simulink model "UPQC_model"  (R2020b)
settings: Solver=FixedStepAuto  StartTime=0.0  StopTime=Tsim  FixedStep=Tsample  MaxStep=Tsample  RelTol=1e-3
values from neighbouring files (symbols this model uses):
  C_parallel_Series = zeros(1,4)    [Netzmodell_Ini_DL.m]    (also in workspace_Ini.mat = [1e-05 1e-05 1e-05 0])
  C_parallel_Shunt = zeros(1,4)    [Netzmodell_Ini_DL.m]    (also in workspace_Ini.mat = [1e-05 1e-05 1e-05 0])
  CC_Ki = 5    [Netzmodell_Ini_DL.m]    (also in workspace_Ini.mat)
  CC_Ki_geg = 5    [Netzmodell_Ini_DL.m]    (also in workspace_Ini.mat)
  CC_Kp = 10    [Netzmodell_Ini_DL.m]    (also in workspace_Ini.mat)
  CC_Kp_geg = 10    [Netzmodell_Ini_DL.m]    (also in workspace_Ini.mat)
  CC_OS =     [workspace_Ini.mat]
  Czk = Szenario.Czk*u    [Netzmodell_Ini_DL.m]    (also in workspace_Ini.mat = 0.003)
  fak_RVC = Szenario.fak_RVC    [Netzmodell_Ini_DL.m]    (also in workspace_Ini.mat = [1 1 1])
  fak_Uns = [1; 1; 1]    [Netzmodell_Ini_DL.m]    (also in workspace_Ini.mat = [1 1 1])
  Flicker_Schaltzeitpunkte_L1 = Schaltzeitpunkte(1,:)    [Netzmodell_Ini_DL.m]    (also in workspace_Ini.mat = 10.5)
  Flicker_Schaltzeitpunkte_L2 = Schaltzeitpunkte(2,:)    [Netzmodell_Ini_DL.m]    (also in workspace_Ini.mat = 10.5)
  Flicker_Schaltzeitpunkte_L3 = Schaltzeitpunkte(3,:)    [Netzmodell_Ini_DL.m]    (also in workspace_Ini.mat = 10.5)
  fs = [f_nom; f_nom; f_nom]    [Netzmodell_Ini_DL.m]    (also in workspace_Ini.mat = [50 50 50])
  fsw = Szenario.fsw*k    [Netzmodell_Ini_DL.m]    (also in workspace_Ini.mat = 20000)
  I_Basis_Ober_L1 = I_Basis_Ober(1)    [Netzmodell_Ini_DL.m]    (also in workspace_Ini.mat = 0)
  I_Basis_Ober_L2 = I_Basis_Ober(2)    [Netzmodell_Ini_DL.m]    (also in workspace_Ini.mat = 0)
  I_Basis_Ober_L3 = I_Basis_Ober(3)    [Netzmodell_Ini_DL.m]    (also in workspace_Ini.mat = 0)
  I_relativ_Ober_L1 = Szenario.I_relativ_Ober_L1    [Netzmodell_Ini_DL.m]    (also in workspace_Ini.mat = [0 100 0 100 100 0 100 100 0 0 0 0 ... (50 elements, 1x50)])
  I_relativ_Ober_L2 = Szenario.I_relativ_Ober_L2    [Netzmodell_Ini_DL.m]    (also in workspace_Ini.mat = [0 100 0 100 100 0 100 100 0 0 0 0 ... (50 elements, 1x50)])
  I_relativ_Ober_L3 = Szenario.I_relativ_Ober_L3    [Netzmodell_Ini_DL.m]    (also in workspace_Ini.mat = [0 100 0 100 100 0 100 100 0 0 0 0 ... (50 elements, 1x50)])
  L_Ausgang_Series = zeros(1,4)    [Netzmodell_Ini_DL.m]    (also in workspace_Ini.mat = [0.00093 0.00093 0.00093 0.00093])
  L_Ausgang_Shunt = zeros(1,4)    [Netzmodell_Ini_DL.m]    (also in workspace_Ini.mat = [0.00093 0.00093 0.00093 0.00093])
  L_Eingang_Series = zeros(1,4)    [Netzmodell_Ini_DL.m]    (also in workspace_Ini.mat = [0.00085 0.00085 0.00085 0.00085])
  L_Eingang_Shunt = zeros(1,4)    [Netzmodell_Ini_DL.m]    (also in workspace_Ini.mat = [0.00085 0.00085 0.00085 0.00085])
  Ls_in = 52.2*u/10    (= 5.22e-06)    [Netzmodell_Ini_DL.m]    (also in workspace_Ini.mat)
  Ltrans = Szenario.Ltrans*m    [Netzmodell_Ini_DL.m]    (also in workspace_Ini.mat = 0.000256)
  OS_off = 6    [Netzmodell_Ini_DL.m]    (also in workspace_Ini.mat)
  OS_on = 1    [Netzmodell_Ini_DL.m]    (also in workspace_Ini.mat)
  Phi_Ober_L1 = Phi_Ober(1)    [Netzmodell_Ini_DL.m]    (also in workspace_Ini.mat = 0)
  Phi_Ober_L2 = Phi_Ober(2)    [Netzmodell_Ini_DL.m]    (also in workspace_Ini.mat = -120)
  Phi_Ober_L3 = Phi_Ober(3)    [Netzmodell_Ini_DL.m]    (also in workspace_Ini.mat = 120)
  Phis = [0; -120; 120]    [Netzmodell_Ini_DL.m]    (also in workspace_Ini.mat = [0 -120 120])
  Pl_Flicker = Pl_Flicker*k    [Netzmodell_Ini_DL.m]    (also in workspace_Ini.mat = [5000 5000 5000])
  Pl_Grund = Szenario.Pl_Grund *k    [Netzmodell_Ini_DL.m]    (also in workspace_Ini.mat = [5 5 5])
  Pl_RVC = Pl_RVC*k    [Netzmodell_Ini_DL.m]    (also in workspace_Ini.mat = [10000 10000 10000])
  Pl_Uns = Pl_Uns*k    [Netzmodell_Ini_DL.m]    (also in workspace_Ini.mat = [25000 10 10])
  Ql_ind_Flicker = Ql_ind_Flicker*k    [Netzmodell_Ini_DL.m]    (also in workspace_Ini.mat = [0 0 0])
  Ql_ind_Grund = Szenario.Ql_ind_Grund*k    [Netzmodell_Ini_DL.m]    (also in workspace_Ini.mat = [0 0 0])
  Ql_ind_RVC = Szenario.Ql_ind_RVC*k    [Netzmodell_Ini_DL.m]    (also in workspace_Ini.mat = [0 0 0])
  Ql_ind_Uns = Ql_ind_Uns*k    [Netzmodell_Ini_DL.m]    (also in workspace_Ini.mat = [0 0 0])
  Ql_kap_Flicker = Ql_kap_Flicker*k    [Netzmodell_Ini_DL.m]    (also in workspace_Ini.mat = [0 0 0])
  Ql_kap_Grund = Szenario.Ql_kap_Grund*k    [Netzmodell_Ini_DL.m]    (also in workspace_Ini.mat = [0 0 0])
  Ql_kap_RVC = Szenario.Ql_kap_RVC*k    [Netzmodell_Ini_DL.m]    (also in workspace_Ini.mat = [0 0 0])
  Ql_kap_Uns = Ql_kap_Uns*k    [Netzmodell_Ini_DL.m]    (also in workspace_Ini.mat = [0 0 0])
  R_Ausgang_Series = zeros(1,4)    [Netzmodell_Ini_DL.m]    (also in workspace_Ini.mat = [0.1 0.1 0.1 0.1])
  R_Ausgang_Shunt = zeros(1,4)    [Netzmodell_Ini_DL.m]    (also in workspace_Ini.mat = [0.1 0.1 0.1 0.1])
  R_Eingang_Series = zeros(1,4)    [Netzmodell_Ini_DL.m]    (also in workspace_Ini.mat = [0.1 0.1 0.1 0.1])
  R_Eingang_Shunt = zeros(1,4)    [Netzmodell_Ini_DL.m]    (also in workspace_Ini.mat = [0.1 0.1 0.1 0.1])
  R_parallel_Series = zeros(1,4)    [Netzmodell_Ini_DL.m]    (also in workspace_Ini.mat = [13 13 13 0])
  R_parallel_Shunt = zeros(1,4)    [Netzmodell_Ini_DL.m]    (also in workspace_Ini.mat = [13 13 13 0])
  R_ZK_Belastung = 20    [Netzmodell_Ini_DL.m]    (also in workspace_Ini.mat)
  Rs_in = 5.2*m/10    (= 0.00052)    [Netzmodell_Ini_DL.m]    (also in workspace_Ini.mat)
  Rtrans = Szenario.Rtrans    [Netzmodell_Ini_DL.m]    (also in workspace_Ini.mat = 0.206)
  RVC_L1_on_off_Zeitpunkte = Szenario.RVC_L1_on_off_Zeitpunkte    [Netzmodell_Ini_DL.m]    (also in workspace_Ini.mat = [10.5 40 10 11 12 13 14 15])
  RVC_L2_on_off_Zeitpunkte = Szenario.RVC_L2_on_off_Zeitpunkte    [Netzmodell_Ini_DL.m]    (also in workspace_Ini.mat = [10.5 40 10 11 12 13 14 15])
  RVC_L3_on_off_Zeitpunkte = Szenario.RVC_L3_on_off_Zeitpunkte    [Netzmodell_Ini_DL.m]    (also in workspace_Ini.mat = [10.5 40 10 11 12 13 14 15])
  RVC_off = 20.5    [Netzmodell_Ini_DL.m]    (also in workspace_Ini.mat)
  RVC_on = 20    [Netzmodell_Ini_DL.m]    (also in workspace_Ini.mat)
  RVC_val = [0.8,0.8,0.8]    [Netzmodell_Ini_DL.m]    (also in workspace_Ini.mat = [0.8 0.8 0.8])
  strans = Szenario.strans    [Netzmodell_Ini_DL.m]    (also in workspace_Ini.mat = 0.25)
  t_breaker_series = tacts    [Netzmodell_Ini_DL.m]    (also in workspace_Ini.mat = 0.5)
  tact = Szenario.tact    [Netzmodell_Ini_DL.m]    (also in workspace_Ini.mat = 0.5)
  tact_OS_Regler = Szenario.tact_OS_Regler    [Netzmodell_Ini_DL.m]    (also in workspace_Ini.mat = 0.5)
  tact_QU = 10    [Netzmodell_Ini_DL.m]    (also in workspace_Ini.mat)
  tacts = Szenario.tacts    [Netzmodell_Ini_DL.m]    (also in workspace_Ini.mat = 0.5)
  Tsample = Szenario.Tsample    [Netzmodell_Ini_DL.m]    (also in workspace_Ini.mat = 5e-06)
  Uns_L1_on_off_Zeitpunkte = Szenario.Uns_L1_on_off_Zeitpunkte    [Netzmodell_Ini_DL.m]    (also in workspace_Ini.mat = [1 6 10 11 12 13 14 15])
  Uns_L2_on_off_Zeitpunkte = Szenario.Uns_L2_on_off_Zeitpunkte    [Netzmodell_Ini_DL.m]    (also in workspace_Ini.mat = [10 30 10 11 12 13 14 15])
  Uns_L3_on_off_Zeitpunkte = Szenario.Uns_L3_on_off_Zeitpunkte    [Netzmodell_Ini_DL.m]    (also in workspace_Ini.mat = [10 30 10 11 12 13 14 15])
  Us = [Us_Amp; Us_Amp; Us_Amp]    [Netzmodell_Ini_DL.m]    (also in workspace_Ini.mat = [326.598632371 326.598632371 326.598632371])
  Us_Amp = sqrt(2)*400/sqrt(3)    [Netzmodell_Ini_DL.m]    (also in workspace_Ini.mat = 326.598632371)
  VC_Ki_gegen = 30    [Netzmodell_Ini_DL.m]    (also in workspace_Ini.mat)
  VC_Ki_gegen_shunt = 15    [Netzmodell_Ini_DL.m]    (also in workspace_Ini.mat)
  VC_Ki_mit = 5    [Netzmodell_Ini_DL.m]    (also in workspace_Ini.mat)
  VC_Kp_gegen = 5    [workspace_Ini.mat]
  VC_Kp_gegen_shunt = 2    [Netzmodell_Ini_DL.m]    (also in workspace_Ini.mat)
  VC_Kp_mit = 10    [Netzmodell_Ini_DL.m]    (also in workspace_Ini.mat)
  VC_ZK_Ki = 5    [Netzmodell_Ini_DL.m]    (also in workspace_Ini.mat)
  VC_ZK_Kp = 0.5    [Netzmodell_Ini_DL.m]    (also in workspace_Ini.mat)
  Vielfache_Ober_L1 = Szenario.Vielfache_Ober_L1    [Netzmodell_Ini_DL.m]    (also in workspace_Ini.mat = [1 2 3 4 5 6 7 8 9 10 11 12 ... (50 elements, 1x50)])
  Vielfache_Ober_L2 = Szenario.Vielfache_Ober_L2    [Netzmodell_Ini_DL.m]    (also in workspace_Ini.mat = [1 2 3 4 5 6 7 8 9 10 11 12 ... (50 elements, 1x50)])
  Vielfache_Ober_L3 = Szenario.Vielfache_Ober_L3    [Netzmodell_Ini_DL.m]    (also in workspace_Ini.mat = [1 2 3 4 5 6 7 8 9 10 11 12 ... (50 elements, 1x50)])
  ZK_Belastung_off = 100    [Netzmodell_Ini_DL.m]    (also in workspace_Ini.mat)
  ZK_Belastung_on = 100    [Netzmodell_Ini_DL.m]    (also in workspace_Ini.mat)
  Zwischenkreisspannung = 700    [Netzmodell_Ini_DL.m]    (also in workspace_Ini.mat)
undefined symbols (not defined in the file or in its folder): LAusgang, RReiheL3
libraries: powerlib x221, powerlib_meascontrol x80, pid_lib x23, eeTransforms x4, eePwmGeneratorTwoLevel x2, dspstat3 x1
(part 8 of 16)

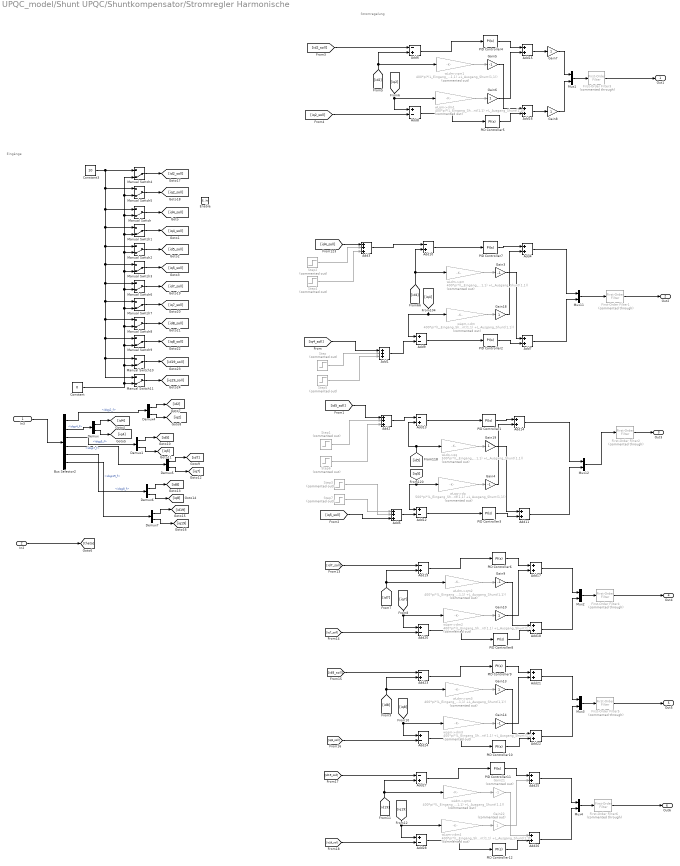
== system UPQC_model/Shunt UPQC/Shuntkompensator/Stromregler Harmonische ==
  note: Eingänge
  note: Stromregelung
  In3 : Inport
  In2 : Inport  Port=2
  Enable : EnablePort
  Add{1..3,5} (4 alike) : Sum  Inputs=+++
  Add{6,10,13,19,23,27} (6 alike) : Sum  Inputs=-+
  Add{4,7,11,14..18,21..22,25..26} (12 alike) : Sum
  Add{8..9,12,20,24,28} (6 alike) : Sum  Inputs=+-
  Bus Selector2 : BusSelector  OutputSignals=idqg2_f,idqp4_f,idqg5_f,idqp7_f,idqg8_f,idqp19_f
  Constant : Constant  Value=0
  Constant3 : Constant  Value=10
  Demux{,1,4..7} (6 alike) : Demux  Outputs=2
  First-Order Filter{1..6} (6 alike) : powerlib_meascontrol/Filters/First-Order Filter  Commented=through  FilterType=Lowpass  Tc=1/(2*25*pi/sqrt(2))  Ts=0  Initialize=off  Vac_Init=[0, 0, 60]  Vdc_Init=0  PlotResponse=off  FreqRange="[0,  30,  1]"
  Gain{6..8,10,13,18..19} (7 alike) : Gain
  Gain{3..5,9,14} (5 alike) : Gain  Gain=-1
  Gain21 : Gain  Commented=on  Gain=-1
  Gain22 : Gain  Commented=on
  Manual Switch{,1..11} (12 alike) : ManualSwitch  CurrentSetting=0
  Mux{1..4,11..12} (6 alike) : Mux  Inputs=2
  PID Controller1 : pid_lib/PID Controller  Controller=PI  Form=Parallel  TimeDomain=Continuous-time  UseExternalTs=off  SampleTime=-1  IntegratorMethod=Forward Euler  FilterMethod=Forward Euler  ControllerParametersSource=internal  P=CC_OS.Kp5  I=CC_OS.Ki5  D=0  UseFilter=on  N=100  TunerSelectOption=Transfer Function Based (PID Tuner App)  InitialConditionSource=internal  InitialConditionForIntegrator=0  InitialConditionForFilter=0  DifferentiatorICPrevScaledInput=0  ExternalReset=none  TrackingMode=off  Kt=1  LimitOutput=off  SatLimitsSource=internal  UpperSaturationLimit=800  LowerSaturationLimit=-800  LinearizeAsGain=on  AntiWindupMode=none  Kb=1  POutMin=[]  POutMax=[]  IOutMin=[]  IOutMax=[]  DOutMin=[]  DOutMax=[]  NOutMin=[]  NOutMax=[]  SumOutMin=[]  SumOutMax=[]  SaturationOutMin=[]  SaturationOutMax=[]  PParamMin=[]  PParamMax=[]  IParamMin=[]  IParamMax=[]  DParamMin=[]  DParamMax=[]  NParamMin=[]  NParamMax=[]  KbParamMin=[]  KbParamMax=[]  KtParamMin=[]  KtParamMax=[]  KbOutMin=[]  KbOutMax=[]  KtOutMin=[]  KtOutMax=[]  IntegratorOutMin=[]  IntegratorOutMax=[]  FilterOutMin=[]  FilterOutMax=[]  SumI1OutMin=[]  SumI1OutMax=[]  SumI2OutMin=[]  SumI2OutMax=[]  SumI3OutMin=[]  SumI3OutMax=[]  SumI4OutMin=[]  SumI4OutMax=[]  SumDOutMin=[]  SumDOutMax=[]  DifferentiatorOutMin=[]  DifferentiatorOutMax=[]  FilterDiffOutCoefMin=[]  FilterDiffOutCoefMax=[]  ReciprocalOutMin=[]  ReciprocalOutMax=[]  SumDenOutMin=[]  SumDenOutMax=[]  SumNumOutMin=[]  SumNumOutMax=[]  DivideOutMin=[]  DivideOutMax=[]  UdiffTsProdOutMin=[]  UdiffTsProdOutMax=[]  NTsProdOutMin=[]  NTsProdOutMax=[]  UintegralTsProdOutMin=[]  UintegralTsProdOutMax=[]  UngainTsProdOutMin=[]  UngainTsProdOutMax=[]  IntegratorContinuousStateAttributes=''  IntegratorStateMustResolveToSignalObject=off  IntegratorRTWStateStorageClass=Auto  FilterContinuousStateAttributes=''  FilterStateMustResolveToSignalObject=off  FilterRTWStateStorageClass=Auto  ParallelPVariant=InternalParameters  IdealPVariant=Disabled  IVariant=InternalParameters  DVariant=Disabled  IntegratorVariant=Continuous  SatVariant=Disabled  AWVariant=Passthrough  PCopyVariant=Disabled  TRVariant=Disabled  FdbkBlocksVariant=Forward  IdealPFdbkVariant=Disabled  SatFdbkVariant=Disabled  DerivativeFilterVariant=Disabled  NVariant=Disabled  NCopyVariant=Disabled_SignalSpec  FilterICVariant=Disabled  IntegratorICVariant=InternalICs  ExternalResetVariant=Disabled  TRSumVariant=Passthrough  SumFdbkVariant=Disabled  SumVariant=Sum_PI  TsampFilterVariant=InternalTs  TsampNgainVariant=Passthrough  TsampIntegralVariant=Passthrough  ExternalSaturationOutDataTypeStr=Inherit: Same as second input
  PID Controller10 : pid_lib/PID Controller  Controller=PI  Form=Parallel  TimeDomain=Continuous-time  UseExternalTs=off  SampleTime=-1  IntegratorMethod=Forward Euler  FilterMethod=Forward Euler  ControllerParametersSource=internal  P=CC_OS.Kp8  I=CC_OS.Ki8  D=0  UseFilter=on  N=100  TunerSelectOption=Transfer Function Based (PID Tuner App)  InitialConditionSource=internal  InitialConditionForIntegrator=0  InitialConditionForFilter=0  DifferentiatorICPrevScaledInput=0  ExternalReset=none  TrackingMode=off  Kt=1  LimitOutput=off  SatLimitsSource=internal  UpperSaturationLimit=800  LowerSaturationLimit=-800  LinearizeAsGain=on  AntiWindupMode=none  Kb=1  POutMin=[]  POutMax=[]  IOutMin=[]  IOutMax=[]  DOutMin=[]  DOutMax=[]  NOutMin=[]  NOutMax=[]  SumOutMin=[]  SumOutMax=[]  SaturationOutMin=[]  SaturationOutMax=[]  PParamMin=[]  PParamMax=[]  IParamMin=[]  IParamMax=[]  DParamMin=[]  DParamMax=[]  NParamMin=[]  NParamMax=[]  KbParamMin=[]  KbParamMax=[]  KtParamMin=[]  KtParamMax=[]  KbOutMin=[]  KbOutMax=[]  KtOutMin=[]  KtOutMax=[]  IntegratorOutMin=[]  IntegratorOutMax=[]  FilterOutMin=[]  FilterOutMax=[]  SumI1OutMin=[]  SumI1OutMax=[]  SumI2OutMin=[]  SumI2OutMax=[]  SumI3OutMin=[]  SumI3OutMax=[]  SumI4OutMin=[]  SumI4OutMax=[]  SumDOutMin=[]  SumDOutMax=[]  DifferentiatorOutMin=[]  DifferentiatorOutMax=[]  FilterDiffOutCoefMin=[]  FilterDiffOutCoefMax=[]  ReciprocalOutMin=[]  ReciprocalOutMax=[]  SumDenOutMin=[]  SumDenOutMax=[]  SumNumOutMin=[]  SumNumOutMax=[]  DivideOutMin=[]  DivideOutMax=[]  UdiffTsProdOutMin=[]  UdiffTsProdOutMax=[]  NTsProdOutMin=[]  NTsProdOutMax=[]  UintegralTsProdOutMin=[]  UintegralTsProdOutMax=[]  UngainTsProdOutMin=[]  UngainTsProdOutMax=[]  IntegratorContinuousStateAttributes=''  IntegratorStateMustResolveToSignalObject=off  IntegratorRTWStateStorageClass=Auto  FilterContinuousStateAttributes=''  FilterStateMustResolveToSignalObject=off  FilterRTWStateStorageClass=Auto  ParallelPVariant=InternalParameters  IdealPVariant=Disabled  IVariant=InternalParameters  DVariant=Disabled  IntegratorVariant=Continuous  SatVariant=Disabled  AWVariant=Passthrough  PCopyVariant=Disabled  TRVariant=Disabled  FdbkBlocksVariant=Forward  IdealPFdbkVariant=Disabled  SatFdbkVariant=Disabled  DerivativeFilterVariant=Disabled  NVariant=Disabled  NCopyVariant=Disabled_SignalSpec  FilterICVariant=Disabled  IntegratorICVariant=InternalICs  ExternalResetVariant=Disabled  TRSumVariant=Passthrough  SumFdbkVariant=Disabled  SumVariant=Sum_PI  TsampFilterVariant=InternalTs  TsampNgainVariant=Passthrough  TsampIntegralVariant=Passthrough  ExternalSaturationOutDataTypeStr=Inherit: Same as second input
  PID Controller11 : pid_lib/PID Controller  Controller=PI  Form=Parallel  TimeDomain=Continuous-time  UseExternalTs=off  SampleTime=-1  IntegratorMethod=Forward Euler  FilterMethod=Forward Euler  ControllerParametersSource=internal  P=CC_OS.Kp19  I=CC_OS.Ki19  D=0  UseFilter=on  N=100  TunerSelectOption=Transfer Function Based (PID Tuner App)  InitialConditionSource=internal  InitialConditionForIntegrator=0  InitialConditionForFilter=0  DifferentiatorICPrevScaledInput=0  ExternalReset=none  TrackingMode=off  Kt=1  LimitOutput=off  SatLimitsSource=internal  UpperSaturationLimit=800  LowerSaturationLimit=-800  LinearizeAsGain=on  AntiWindupMode=none  Kb=1  POutMin=[]  POutMax=[]  IOutMin=[]  IOutMax=[]  DOutMin=[]  DOutMax=[]  NOutMin=[]  NOutMax=[]  SumOutMin=[]  SumOutMax=[]  SaturationOutMin=[]  SaturationOutMax=[]  PParamMin=[]  PParamMax=[]  IParamMin=[]  IParamMax=[]  DParamMin=[]  DParamMax=[]  NParamMin=[]  NParamMax=[]  KbParamMin=[]  KbParamMax=[]  KtParamMin=[]  KtParamMax=[]  KbOutMin=[]  KbOutMax=[]  KtOutMin=[]  KtOutMax=[]  IntegratorOutMin=[]  IntegratorOutMax=[]  FilterOutMin=[]  FilterOutMax=[]  SumI1OutMin=[]  SumI1OutMax=[]  SumI2OutMin=[]  SumI2OutMax=[]  SumI3OutMin=[]  SumI3OutMax=[]  SumI4OutMin=[]  SumI4OutMax=[]  SumDOutMin=[]  SumDOutMax=[]  DifferentiatorOutMin=[]  DifferentiatorOutMax=[]  FilterDiffOutCoefMin=[]  FilterDiffOutCoefMax=[]  ReciprocalOutMin=[]  ReciprocalOutMax=[]  SumDenOutMin=[]  SumDenOutMax=[]  SumNumOutMin=[]  SumNumOutMax=[]  DivideOutMin=[]  DivideOutMax=[]  UdiffTsProdOutMin=[]  UdiffTsProdOutMax=[]  NTsProdOutMin=[]  NTsProdOutMax=[]  UintegralTsProdOutMin=[]  UintegralTsProdOutMax=[]  UngainTsProdOutMin=[]  UngainTsProdOutMax=[]  IntegratorContinuousStateAttributes=''  IntegratorStateMustResolveToSignalObject=off  IntegratorRTWStateStorageClass=Auto  FilterContinuousStateAttributes=''  FilterStateMustResolveToSignalObject=off  FilterRTWStateStorageClass=Auto  ParallelPVariant=InternalParameters  IdealPVariant=Disabled  IVariant=InternalParameters  DVariant=Disabled  IntegratorVariant=Continuous  SatVariant=Disabled  AWVariant=Passthrough  PCopyVariant=Disabled  TRVariant=Disabled  FdbkBlocksVariant=Forward  IdealPFdbkVariant=Disabled  SatFdbkVariant=Disabled  DerivativeFilterVariant=Disabled  NVariant=Disabled  NCopyVariant=Disabled_SignalSpec  FilterICVariant=Disabled  IntegratorICVariant=InternalICs  ExternalResetVariant=Disabled  TRSumVariant=Passthrough  SumFdbkVariant=Disabled  SumVariant=Sum_PI  TsampFilterVariant=InternalTs  TsampNgainVariant=Passthrough  TsampIntegralVariant=Passthrough  ExternalSaturationOutDataTypeStr=Inherit: Same as second input
  PID Controller12 : pid_lib/PID Controller  Controller=PI  Form=Parallel  TimeDomain=Continuous-time  UseExternalTs=off  SampleTime=-1  IntegratorMethod=Forward Euler  FilterMethod=Forward Euler  ControllerParametersSource=internal  P=CC_OS.Kp19  I=CC_OS.Ki19  D=0  UseFilter=on  N=100  TunerSelectOption=Transfer Function Based (PID Tuner App)  InitialConditionSource=internal  InitialConditionForIntegrator=0  InitialConditionForFilter=0  DifferentiatorICPrevScaledInput=0  ExternalReset=none  TrackingMode=off  Kt=1  LimitOutput=off  SatLimitsSource=internal  UpperSaturationLimit=800  LowerSaturationLimit=-800  LinearizeAsGain=on  AntiWindupMode=none  Kb=1  POutMin=[]  POutMax=[]  IOutMin=[]  IOutMax=[]  DOutMin=[]  DOutMax=[]  NOutMin=[]  NOutMax=[]  SumOutMin=[]  SumOutMax=[]  SaturationOutMin=[]  SaturationOutMax=[]  PParamMin=[]  PParamMax=[]  IParamMin=[]  IParamMax=[]  DParamMin=[]  DParamMax=[]  NParamMin=[]  NParamMax=[]  KbParamMin=[]  KbParamMax=[]  KtParamMin=[]  KtParamMax=[]  KbOutMin=[]  KbOutMax=[]  KtOutMin=[]  KtOutMax=[]  IntegratorOutMin=[]  IntegratorOutMax=[]  FilterOutMin=[]  FilterOutMax=[]  SumI1OutMin=[]  SumI1OutMax=[]  SumI2OutMin=[]  SumI2OutMax=[]  SumI3OutMin=[]  SumI3OutMax=[]  SumI4OutMin=[]  SumI4OutMax=[]  SumDOutMin=[]  SumDOutMax=[]  DifferentiatorOutMin=[]  DifferentiatorOutMax=[]  FilterDiffOutCoefMin=[]  FilterDiffOutCoefMax=[]  ReciprocalOutMin=[]  ReciprocalOutMax=[]  SumDenOutMin=[]  SumDenOutMax=[]  SumNumOutMin=[]  SumNumOutMax=[]  DivideOutMin=[]  DivideOutMax=[]  UdiffTsProdOutMin=[]  UdiffTsProdOutMax=[]  NTsProdOutMin=[]  NTsProdOutMax=[]  UintegralTsProdOutMin=[]  UintegralTsProdOutMax=[]  UngainTsProdOutMin=[]  UngainTsProdOutMax=[]  IntegratorContinuousStateAttributes=''  IntegratorStateMustResolveToSignalObject=off  IntegratorRTWStateStorageClass=Auto  FilterContinuousStateAttributes=''  FilterStateMustResolveToSignalObject=off  FilterRTWStateStorageClass=Auto  ParallelPVariant=InternalParameters  IdealPVariant=Disabled  IVariant=InternalParameters  DVariant=Disabled  IntegratorVariant=Continuous  SatVariant=Disabled  AWVariant=Passthrough  PCopyVariant=Disabled  TRVariant=Disabled  FdbkBlocksVariant=Forward  IdealPFdbkVariant=Disabled  SatFdbkVariant=Disabled  DerivativeFilterVariant=Disabled  NVariant=Disabled  NCopyVariant=Disabled_SignalSpec  FilterICVariant=Disabled  IntegratorICVariant=InternalICs  ExternalResetVariant=Disabled  TRSumVariant=Passthrough  SumFdbkVariant=Disabled  SumVariant=Sum_PI  TsampFilterVariant=InternalTs  TsampNgainVariant=Passthrough  TsampIntegralVariant=Passthrough  ExternalSaturationOutDataTypeStr=Inherit: Same as second input
  PID Controller2 : pid_lib/PID Controller  Controller=PI  Form=Parallel  TimeDomain=Continuous-time  UseExternalTs=off  SampleTime=-1  IntegratorMethod=Forward Euler  FilterMethod=Forward Euler  ControllerParametersSource=internal  P=CC_OS.Kp4  I=CC_OS.Ki4  D=0  UseFilter=on  N=100  TunerSelectOption=Transfer Function Based (PID Tuner App)  InitialConditionSource=internal  InitialConditionForIntegrator=0  InitialConditionForFilter=0  DifferentiatorICPrevScaledInput=0  ExternalReset=none  TrackingMode=off  Kt=1  LimitOutput=off  SatLimitsSource=internal  UpperSaturationLimit=800  LowerSaturationLimit=-800  LinearizeAsGain=on  AntiWindupMode=none  Kb=1  POutMin=[]  POutMax=[]  IOutMin=[]  IOutMax=[]  DOutMin=[]  DOutMax=[]  NOutMin=[]  NOutMax=[]  SumOutMin=[]  SumOutMax=[]  SaturationOutMin=[]  SaturationOutMax=[]  PParamMin=[]  PParamMax=[]  IParamMin=[]  IParamMax=[]  DParamMin=[]  DParamMax=[]  NParamMin=[]  NParamMax=[]  KbParamMin=[]  KbParamMax=[]  KtParamMin=[]  KtParamMax=[]  KbOutMin=[]  KbOutMax=[]  KtOutMin=[]  KtOutMax=[]  IntegratorOutMin=[]  IntegratorOutMax=[]  FilterOutMin=[]  FilterOutMax=[]  SumI1OutMin=[]  SumI1OutMax=[]  SumI2OutMin=[]  SumI2OutMax=[]  SumI3OutMin=[]  SumI3OutMax=[]  SumI4OutMin=[]  SumI4OutMax=[]  SumDOutMin=[]  SumDOutMax=[]  DifferentiatorOutMin=[]  DifferentiatorOutMax=[]  FilterDiffOutCoefMin=[]  FilterDiffOutCoefMax=[]  ReciprocalOutMin=[]  ReciprocalOutMax=[]  SumDenOutMin=[]  SumDenOutMax=[]  SumNumOutMin=[]  SumNumOutMax=[]  DivideOutMin=[]  DivideOutMax=[]  UdiffTsProdOutMin=[]  UdiffTsProdOutMax=[]  NTsProdOutMin=[]  NTsProdOutMax=[]  UintegralTsProdOutMin=[]  UintegralTsProdOutMax=[]  UngainTsProdOutMin=[]  UngainTsProdOutMax=[]  IntegratorContinuousStateAttributes=''  IntegratorStateMustResolveToSignalObject=off  IntegratorRTWStateStorageClass=Auto  FilterContinuousStateAttributes=''  FilterStateMustResolveToSignalObject=off  FilterRTWStateStorageClass=Auto  ParallelPVariant=InternalParameters  IdealPVariant=Disabled  IVariant=InternalParameters  DVariant=Disabled  IntegratorVariant=Continuous  SatVariant=Disabled  AWVariant=Passthrough  PCopyVariant=Disabled  TRVariant=Disabled  FdbkBlocksVariant=Forward  IdealPFdbkVariant=Disabled  SatFdbkVariant=Disabled  DerivativeFilterVariant=Disabled  NVariant=Disabled  NCopyVariant=Disabled_SignalSpec  FilterICVariant=Disabled  IntegratorICVariant=InternalICs  ExternalResetVariant=Disabled  TRSumVariant=Passthrough  SumFdbkVariant=Disabled  SumVariant=Sum_PI  TsampFilterVariant=InternalTs  TsampNgainVariant=Passthrough  TsampIntegralVariant=Passthrough  ExternalSaturationOutDataTypeStr=Inherit: Same as second input
  PID Controller3 : pid_lib/PID Controller  Controller=PI  Form=Parallel  TimeDomain=Continuous-time  UseExternalTs=off  SampleTime=-1  IntegratorMethod=Forward Euler  FilterMethod=Forward Euler  ControllerParametersSource=internal  P=CC_OS.Kp5  I=CC_OS.Ki5  D=0  UseFilter=on  N=100  TunerSelectOption=Transfer Function Based (PID Tuner App)  InitialConditionSource=internal  InitialConditionForIntegrator=0  InitialConditionForFilter=0  DifferentiatorICPrevScaledInput=0  ExternalReset=none  TrackingMode=off  Kt=1  LimitOutput=off  SatLimitsSource=internal  UpperSaturationLimit=800  LowerSaturationLimit=-800  LinearizeAsGain=on  AntiWindupMode=none  Kb=1  POutMin=[]  POutMax=[]  IOutMin=[]  IOutMax=[]  DOutMin=[]  DOutMax=[]  NOutMin=[]  NOutMax=[]  SumOutMin=[]  SumOutMax=[]  SaturationOutMin=[]  SaturationOutMax=[]  PParamMin=[]  PParamMax=[]  IParamMin=[]  IParamMax=[]  DParamMin=[]  DParamMax=[]  NParamMin=[]  NParamMax=[]  KbParamMin=[]  KbParamMax=[]  KtParamMin=[]  KtParamMax=[]  KbOutMin=[]  KbOutMax=[]  KtOutMin=[]  KtOutMax=[]  IntegratorOutMin=[]  IntegratorOutMax=[]  FilterOutMin=[]  FilterOutMax=[]  SumI1OutMin=[]  SumI1OutMax=[]  SumI2OutMin=[]  SumI2OutMax=[]  SumI3OutMin=[]  SumI3OutMax=[]  SumI4OutMin=[]  SumI4OutMax=[]  SumDOutMin=[]  SumDOutMax=[]  DifferentiatorOutMin=[]  DifferentiatorOutMax=[]  FilterDiffOutCoefMin=[]  FilterDiffOutCoefMax=[]  ReciprocalOutMin=[]  ReciprocalOutMax=[]  SumDenOutMin=[]  SumDenOutMax=[]  SumNumOutMin=[]  SumNumOutMax=[]  DivideOutMin=[]  DivideOutMax=[]  UdiffTsProdOutMin=[]  UdiffTsProdOutMax=[]  NTsProdOutMin=[]  NTsProdOutMax=[]  UintegralTsProdOutMin=[]  UintegralTsProdOutMax=[]  UngainTsProdOutMin=[]  UngainTsProdOutMax=[]  IntegratorContinuousStateAttributes=''  IntegratorStateMustResolveToSignalObject=off  IntegratorRTWStateStorageClass=Auto  FilterContinuousStateAttributes=''  FilterStateMustResolveToSignalObject=off  FilterRTWStateStorageClass=Auto  ParallelPVariant=InternalParameters  IdealPVariant=Disabled  IVariant=InternalParameters  DVariant=Disabled  IntegratorVariant=Continuous  SatVariant=Disabled  AWVariant=Passthrough  PCopyVariant=Disabled  TRVariant=Disabled  FdbkBlocksVariant=Forward  IdealPFdbkVariant=Disabled  SatFdbkVariant=Disabled  DerivativeFilterVariant=Disabled  NVariant=Disabled  NCopyVariant=Disabled_SignalSpec  FilterICVariant=Disabled  IntegratorICVariant=InternalICs  ExternalResetVariant=Disabled  TRSumVariant=Passthrough  SumFdbkVariant=Disabled  SumVariant=Sum_PI  TsampFilterVariant=InternalTs  TsampNgainVariant=Passthrough  TsampIntegralVariant=Passthrough  ExternalSaturationOutDataTypeStr=Inherit: Same as second input
  PID Controller4 : pid_lib/PID Controller  Controller=PI  Form=Parallel  TimeDomain=Continuous-time  UseExternalTs=off  SampleTime=-1  IntegratorMethod=Forward Euler  FilterMethod=Forward Euler  ControllerParametersSource=internal  P=CC_OS.Kp2  I=CC_OS.Ki2  D=0  UseFilter=on  N=100  TunerSelectOption=Transfer Function Based (PID Tuner App)  InitialConditionSource=internal  InitialConditionForIntegrator=0  InitialConditionForFilter=0  DifferentiatorICPrevScaledInput=0  ExternalReset=none  TrackingMode=off  Kt=1  LimitOutput=off  SatLimitsSource=internal  UpperSaturationLimit=800  LowerSaturationLimit=-800  LinearizeAsGain=on  AntiWindupMode=none  Kb=1  POutMin=[]  POutMax=[]  IOutMin=[]  IOutMax=[]  DOutMin=[]  DOutMax=[]  NOutMin=[]  NOutMax=[]  SumOutMin=[]  SumOutMax=[]  SaturationOutMin=[]  SaturationOutMax=[]  PParamMin=[]  PParamMax=[]  IParamMin=[]  IParamMax=[]  DParamMin=[]  DParamMax=[]  NParamMin=[]  NParamMax=[]  KbParamMin=[]  KbParamMax=[]  KtParamMin=[]  KtParamMax=[]  KbOutMin=[]  KbOutMax=[]  KtOutMin=[]  KtOutMax=[]  IntegratorOutMin=[]  IntegratorOutMax=[]  FilterOutMin=[]  FilterOutMax=[]  SumI1OutMin=[]  SumI1OutMax=[]  SumI2OutMin=[]  SumI2OutMax=[]  SumI3OutMin=[]  SumI3OutMax=[]  SumI4OutMin=[]  SumI4OutMax=[]  SumDOutMin=[]  SumDOutMax=[]  DifferentiatorOutMin=[]  DifferentiatorOutMax=[]  FilterDiffOutCoefMin=[]  FilterDiffOutCoefMax=[]  ReciprocalOutMin=[]  ReciprocalOutMax=[]  SumDenOutMin=[]  SumDenOutMax=[]  SumNumOutMin=[]  SumNumOutMax=[]  DivideOutMin=[]  DivideOutMax=[]  UdiffTsProdOutMin=[]  UdiffTsProdOutMax=[]  NTsProdOutMin=[]  NTsProdOutMax=[]  UintegralTsProdOutMin=[]  UintegralTsProdOutMax=[]  UngainTsProdOutMin=[]  UngainTsProdOutMax=[]  IntegratorContinuousStateAttributes=''  IntegratorStateMustResolveToSignalObject=off  IntegratorRTWStateStorageClass=Auto  FilterContinuousStateAttributes=''  FilterStateMustResolveToSignalObject=off  FilterRTWStateStorageClass=Auto  ParallelPVariant=InternalParameters  IdealPVariant=Disabled  IVariant=InternalParameters  DVariant=Disabled  IntegratorVariant=Continuous  SatVariant=Disabled  AWVariant=Passthrough  PCopyVariant=Disabled  TRVariant=Disabled  FdbkBlocksVariant=Forward  IdealPFdbkVariant=Disabled  SatFdbkVariant=Disabled  DerivativeFilterVariant=Disabled  NVariant=Disabled  NCopyVariant=Disabled_SignalSpec  FilterICVariant=Disabled  IntegratorICVariant=InternalICs  ExternalResetVariant=Disabled  TRSumVariant=Passthrough  SumFdbkVariant=Disabled  SumVariant=Sum_PI  TsampFilterVariant=InternalTs  TsampNgainVariant=Passthrough  TsampIntegralVariant=Passthrough  ExternalSaturationOutDataTypeStr=Inherit: Same as second input
  PID Controller5 : pid_lib/PID Controller  Controller=PI  Form=Parallel  TimeDomain=Continuous-time  UseExternalTs=off  SampleTime=-1  IntegratorMethod=Forward Euler  FilterMethod=Forward Euler  ControllerParametersSource=internal  P=CC_OS.Kp2  I=CC_OS.Ki2  D=0  UseFilter=on  N=100  TunerSelectOption=Transfer Function Based (PID Tuner App)  InitialConditionSource=internal  InitialConditionForIntegrator=0  InitialConditionForFilter=0  DifferentiatorICPrevScaledInput=0  ExternalReset=none  TrackingMode=off  Kt=1  LimitOutput=off  SatLimitsSource=internal  UpperSaturationLimit=800  LowerSaturationLimit=-800  LinearizeAsGain=on  AntiWindupMode=none  Kb=1  POutMin=[]  POutMax=[]  IOutMin=[]  IOutMax=[]  DOutMin=[]  DOutMax=[]  NOutMin=[]  NOutMax=[]  SumOutMin=[]  SumOutMax=[]  SaturationOutMin=[]  SaturationOutMax=[]  PParamMin=[]  PParamMax=[]  IParamMin=[]  IParamMax=[]  DParamMin=[]  DParamMax=[]  NParamMin=[]  NParamMax=[]  KbParamMin=[]  KbParamMax=[]  KtParamMin=[]  KtParamMax=[]  KbOutMin=[]  KbOutMax=[]  KtOutMin=[]  KtOutMax=[]  IntegratorOutMin=[]  IntegratorOutMax=[]  FilterOutMin=[]  FilterOutMax=[]  SumI1OutMin=[]  SumI1OutMax=[]  SumI2OutMin=[]  SumI2OutMax=[]  SumI3OutMin=[]  SumI3OutMax=[]  SumI4OutMin=[]  SumI4OutMax=[]  SumDOutMin=[]  SumDOutMax=[]  DifferentiatorOutMin=[]  DifferentiatorOutMax=[]  FilterDiffOutCoefMin=[]  FilterDiffOutCoefMax=[]  ReciprocalOutMin=[]  ReciprocalOutMax=[]  SumDenOutMin=[]  SumDenOutMax=[]  SumNumOutMin=[]  SumNumOutMax=[]  DivideOutMin=[]  DivideOutMax=[]  UdiffTsProdOutMin=[]  UdiffTsProdOutMax=[]  NTsProdOutMin=[]  NTsProdOutMax=[]  UintegralTsProdOutMin=[]  UintegralTsProdOutMax=[]  UngainTsProdOutMin=[]  UngainTsProdOutMax=[]  IntegratorContinuousStateAttributes=''  IntegratorStateMustResolveToSignalObject=off  IntegratorRTWStateStorageClass=Auto  FilterContinuousStateAttributes=''  FilterStateMustResolveToSignalObject=off  FilterRTWStateStorageClass=Auto  ParallelPVariant=InternalParameters  IdealPVariant=Disabled  IVariant=InternalParameters  DVariant=Disabled  IntegratorVariant=Continuous  SatVariant=Disabled  AWVariant=Passthrough  PCopyVariant=Disabled  TRVariant=Disabled  FdbkBlocksVariant=Forward  IdealPFdbkVariant=Disabled  SatFdbkVariant=Disabled  DerivativeFilterVariant=Disabled  NVariant=Disabled  NCopyVariant=Disabled_SignalSpec  FilterICVariant=Disabled  IntegratorICVariant=InternalICs  ExternalResetVariant=Disabled  TRSumVariant=Passthrough  SumFdbkVariant=Disabled  SumVariant=Sum_PI  TsampFilterVariant=InternalTs  TsampNgainVariant=Passthrough  TsampIntegralVariant=Passthrough  ExternalSaturationOutDataTypeStr=Inherit: Same as second input
  PID Controller6 : pid_lib/PID Controller  Controller=PI  Form=Parallel  TimeDomain=Continuous-time  UseExternalTs=off  SampleTime=-1  IntegratorMethod=Forward Euler  FilterMethod=Forward Euler  ControllerParametersSource=internal  P=CC_OS.Kp7  I=CC_OS.Ki7  D=0  UseFilter=on  N=100  TunerSelectOption=Transfer Function Based (PID Tuner App)  InitialConditionSource=internal  InitialConditionForIntegrator=0  InitialConditionForFilter=0  DifferentiatorICPrevScaledInput=0  ExternalReset=none  TrackingMode=off  Kt=1  LimitOutput=off  SatLimitsSource=internal  UpperSaturationLimit=800  LowerSaturationLimit=-800  LinearizeAsGain=on  AntiWindupMode=none  Kb=1  POutMin=[]  POutMax=[]  IOutMin=[]  IOutMax=[]  DOutMin=[]  DOutMax=[]  NOutMin=[]  NOutMax=[]  SumOutMin=[]  SumOutMax=[]  SaturationOutMin=[]  SaturationOutMax=[]  PParamMin=[]  PParamMax=[]  IParamMin=[]  IParamMax=[]  DParamMin=[]  DParamMax=[]  NParamMin=[]  NParamMax=[]  KbParamMin=[]  KbParamMax=[]  KtParamMin=[]  KtParamMax=[]  KbOutMin=[]  KbOutMax=[]  KtOutMin=[]  KtOutMax=[]  IntegratorOutMin=[]  IntegratorOutMax=[]  FilterOutMin=[]  FilterOutMax=[]  SumI1OutMin=[]  SumI1OutMax=[]  SumI2OutMin=[]  SumI2OutMax=[]  SumI3OutMin=[]  SumI3OutMax=[]  SumI4OutMin=[]  SumI4OutMax=[]  SumDOutMin=[]  SumDOutMax=[]  DifferentiatorOutMin=[]  DifferentiatorOutMax=[]  FilterDiffOutCoefMin=[]  FilterDiffOutCoefMax=[]  ReciprocalOutMin=[]  ReciprocalOutMax=[]  SumDenOutMin=[]  SumDenOutMax=[]  SumNumOutMin=[]  SumNumOutMax=[]  DivideOutMin=[]  DivideOutMax=[]  UdiffTsProdOutMin=[]  UdiffTsProdOutMax=[]  NTsProdOutMin=[]  NTsProdOutMax=[]  UintegralTsProdOutMin=[]  UintegralTsProdOutMax=[]  UngainTsProdOutMin=[]  UngainTsProdOutMax=[]  IntegratorContinuousStateAttributes=''  IntegratorStateMustResolveToSignalObject=off  IntegratorRTWStateStorageClass=Auto  FilterContinuousStateAttributes=''  FilterStateMustResolveToSignalObject=off  FilterRTWStateStorageClass=Auto  ParallelPVariant=InternalParameters  IdealPVariant=Disabled  IVariant=InternalParameters  DVariant=Disabled  IntegratorVariant=Continuous  SatVariant=Disabled  AWVariant=Passthrough  PCopyVariant=Disabled  TRVariant=Disabled  FdbkBlocksVariant=Forward  IdealPFdbkVariant=Disabled  SatFdbkVariant=Disabled  DerivativeFilterVariant=Disabled  NVariant=Disabled  NCopyVariant=Disabled_SignalSpec  FilterICVariant=Disabled  IntegratorICVariant=InternalICs  ExternalResetVariant=Disabled  TRSumVariant=Passthrough  SumFdbkVariant=Disabled  SumVariant=Sum_PI  TsampFilterVariant=InternalTs  TsampNgainVariant=Passthrough  TsampIntegralVariant=Passthrough  ExternalSaturationOutDataTypeStr=Inherit: Same as second input
  PID Controller7 : pid_lib/PID Controller  Controller=PI  Form=Parallel  TimeDomain=Continuous-time  UseExternalTs=off  SampleTime=-1  IntegratorMethod=Forward Euler  FilterMethod=Forward Euler  ControllerParametersSource=internal  P=CC_OS.Kp4  I=CC_OS.Ki4  D=0  UseFilter=on  N=100  TunerSelectOption=Transfer Function Based (PID Tuner App)  InitialConditionSource=internal  InitialConditionForIntegrator=0  InitialConditionForFilter=0  DifferentiatorICPrevScaledInput=0  ExternalReset=none  TrackingMode=off  Kt=1  LimitOutput=off  SatLimitsSource=internal  UpperSaturationLimit=800  LowerSaturationLimit=-800  LinearizeAsGain=on  AntiWindupMode=none  Kb=1  POutMin=[]  POutMax=[]  IOutMin=[]  IOutMax=[]  DOutMin=[]  DOutMax=[]  NOutMin=[]  NOutMax=[]  SumOutMin=[]  SumOutMax=[]  SaturationOutMin=[]  SaturationOutMax=[]  PParamMin=[]  PParamMax=[]  IParamMin=[]  IParamMax=[]  DParamMin=[]  DParamMax=[]  NParamMin=[]  NParamMax=[]  KbParamMin=[]  KbParamMax=[]  KtParamMin=[]  KtParamMax=[]  KbOutMin=[]  KbOutMax=[]  KtOutMin=[]  KtOutMax=[]  IntegratorOutMin=[]  IntegratorOutMax=[]  FilterOutMin=[]  FilterOutMax=[]  SumI1OutMin=[]  SumI1OutMax=[]  SumI2OutMin=[]  SumI2OutMax=[]  SumI3OutMin=[]  SumI3OutMax=[]  SumI4OutMin=[]  SumI4OutMax=[]  SumDOutMin=[]  SumDOutMax=[]  DifferentiatorOutMin=[]  DifferentiatorOutMax=[]  FilterDiffOutCoefMin=[]  FilterDiffOutCoefMax=[]  ReciprocalOutMin=[]  ReciprocalOutMax=[]  SumDenOutMin=[]  SumDenOutMax=[]  SumNumOutMin=[]  SumNumOutMax=[]  DivideOutMin=[]  DivideOutMax=[]  UdiffTsProdOutMin=[]  UdiffTsProdOutMax=[]  NTsProdOutMin=[]  NTsProdOutMax=[]  UintegralTsProdOutMin=[]  UintegralTsProdOutMax=[]  UngainTsProdOutMin=[]  UngainTsProdOutMax=[]  IntegratorContinuousStateAttributes=''  IntegratorStateMustResolveToSignalObject=off  IntegratorRTWStateStorageClass=Auto  FilterContinuousStateAttributes=''  FilterStateMustResolveToSignalObject=off  FilterRTWStateStorageClass=Auto  ParallelPVariant=InternalParameters  IdealPVariant=Disabled  IVariant=InternalParameters  DVariant=Disabled  IntegratorVariant=Continuous  SatVariant=Disabled  AWVariant=Passthrough  PCopyVariant=Disabled  TRVariant=Disabled  FdbkBlocksVariant=Forward  IdealPFdbkVariant=Disabled  SatFdbkVariant=Disabled  DerivativeFilterVariant=Disabled  NVariant=Disabled  NCopyVariant=Disabled_SignalSpec  FilterICVariant=Disabled  IntegratorICVariant=InternalICs  ExternalResetVariant=Disabled  TRSumVariant=Passthrough  SumFdbkVariant=Disabled  SumVariant=Sum_PI  TsampFilterVariant=InternalTs  TsampNgainVariant=Passthrough  TsampIntegralVariant=Passthrough  ExternalSaturationOutDataTypeStr=Inherit: Same as second input
  PID Controller8 : pid_lib/PID Controller  Controller=PI  Form=Parallel  TimeDomain=Continuous-time  UseExternalTs=off  SampleTime=-1  IntegratorMethod=Forward Euler  FilterMethod=Forward Euler  ControllerParametersSource=internal  P=CC_OS.Kp7  I=CC_OS.Ki7  D=0  UseFilter=on  N=100  TunerSelectOption=Transfer Function Based (PID Tuner App)  InitialConditionSource=internal  InitialConditionForIntegrator=0  InitialConditionForFilter=0  DifferentiatorICPrevScaledInput=0  ExternalReset=none  TrackingMode=off  Kt=1  LimitOutput=off  SatLimitsSource=internal  UpperSaturationLimit=800  LowerSaturationLimit=-800  LinearizeAsGain=on  AntiWindupMode=none  Kb=1  POutMin=[]  POutMax=[]  IOutMin=[]  IOutMax=[]  DOutMin=[]  DOutMax=[]  NOutMin=[]  NOutMax=[]  SumOutMin=[]  SumOutMax=[]  SaturationOutMin=[]  SaturationOutMax=[]  PParamMin=[]  PParamMax=[]  IParamMin=[]  IParamMax=[]  DParamMin=[]  DParamMax=[]  NParamMin=[]  NParamMax=[]  KbParamMin=[]  KbParamMax=[]  KtParamMin=[]  KtParamMax=[]  KbOutMin=[]  KbOutMax=[]  KtOutMin=[]  KtOutMax=[]  IntegratorOutMin=[]  IntegratorOutMax=[]  FilterOutMin=[]  FilterOutMax=[]  SumI1OutMin=[]  SumI1OutMax=[]  SumI2OutMin=[]  SumI2OutMax=[]  SumI3OutMin=[]  SumI3OutMax=[]  SumI4OutMin=[]  SumI4OutMax=[]  SumDOutMin=[]  SumDOutMax=[]  DifferentiatorOutMin=[]  DifferentiatorOutMax=[]  FilterDiffOutCoefMin=[]  FilterDiffOutCoefMax=[]  ReciprocalOutMin=[]  ReciprocalOutMax=[]  SumDenOutMin=[]  SumDenOutMax=[]  SumNumOutMin=[]  SumNumOutMax=[]  DivideOutMin=[]  DivideOutMax=[]  UdiffTsProdOutMin=[]  UdiffTsProdOutMax=[]  NTsProdOutMin=[]  NTsProdOutMax=[]  UintegralTsProdOutMin=[]  UintegralTsProdOutMax=[]  UngainTsProdOutMin=[]  UngainTsProdOutMax=[]  IntegratorContinuousStateAttributes=''  IntegratorStateMustResolveToSignalObject=off  IntegratorRTWStateStorageClass=Auto  FilterContinuousStateAttributes=''  FilterStateMustResolveToSignalObject=off  FilterRTWStateStorageClass=Auto  ParallelPVariant=InternalParameters  IdealPVariant=Disabled  IVariant=InternalParameters  DVariant=Disabled  IntegratorVariant=Continuous  SatVariant=Disabled  AWVariant=Passthrough  PCopyVariant=Disabled  TRVariant=Disabled  FdbkBlocksVariant=Forward  IdealPFdbkVariant=Disabled  SatFdbkVariant=Disabled  DerivativeFilterVariant=Disabled  NVariant=Disabled  NCopyVariant=Disabled_SignalSpec  FilterICVariant=Disabled  IntegratorICVariant=InternalICs  ExternalResetVariant=Disabled  TRSumVariant=Passthrough  SumFdbkVariant=Disabled  SumVariant=Sum_PI  TsampFilterVariant=InternalTs  TsampNgainVariant=Passthrough  TsampIntegralVariant=Passthrough  ExternalSaturationOutDataTypeStr=Inherit: Same as second input
  PID Controller9 : pid_lib/PID Controller  Controller=PI  Form=Parallel  TimeDomain=Continuous-time  UseExternalTs=off  SampleTime=-1  IntegratorMethod=Forward Euler  FilterMethod=Forward Euler  ControllerParametersSource=internal  P=CC_OS.Kp8  I=CC_OS.Ki8  D=0  UseFilter=on  N=100  TunerSelectOption=Transfer Function Based (PID Tuner App)  InitialConditionSource=internal  InitialConditionForIntegrator=0  InitialConditionForFilter=0  DifferentiatorICPrevScaledInput=0  ExternalReset=none  TrackingMode=off  Kt=1  LimitOutput=off  SatLimitsSource=internal  UpperSaturationLimit=800  LowerSaturationLimit=-800  LinearizeAsGain=on  AntiWindupMode=none  Kb=1  POutMin=[]  POutMax=[]  IOutMin=[]  IOutMax=[]  DOutMin=[]  DOutMax=[]  NOutMin=[]  NOutMax=[]  SumOutMin=[]  SumOutMax=[]  SaturationOutMin=[]  SaturationOutMax=[]  PParamMin=[]  PParamMax=[]  IParamMin=[]  IParamMax=[]  DParamMin=[]  DParamMax=[]  NParamMin=[]  NParamMax=[]  KbParamMin=[]  KbParamMax=[]  KtParamMin=[]  KtParamMax=[]  KbOutMin=[]  KbOutMax=[]  KtOutMin=[]  KtOutMax=[]  IntegratorOutMin=[]  IntegratorOutMax=[]  FilterOutMin=[]  FilterOutMax=[]  SumI1OutMin=[]  SumI1OutMax=[]  SumI2OutMin=[]  SumI2OutMax=[]  SumI3OutMin=[]  SumI3OutMax=[]  SumI4OutMin=[]  SumI4OutMax=[]  SumDOutMin=[]  SumDOutMax=[]  DifferentiatorOutMin=[]  DifferentiatorOutMax=[]  FilterDiffOutCoefMin=[]  FilterDiffOutCoefMax=[]  ReciprocalOutMin=[]  ReciprocalOutMax=[]  SumDenOutMin=[]  SumDenOutMax=[]  SumNumOutMin=[]  SumNumOutMax=[]  DivideOutMin=[]  DivideOutMax=[]  UdiffTsProdOutMin=[]  UdiffTsProdOutMax=[]  NTsProdOutMin=[]  NTsProdOutMax=[]  UintegralTsProdOutMin=[]  UintegralTsProdOutMax=[]  UngainTsProdOutMin=[]  UngainTsProdOutMax=[]  IntegratorContinuousStateAttributes=''  IntegratorStateMustResolveToSignalObject=off  IntegratorRTWStateStorageClass=Auto  FilterContinuousStateAttributes=''  FilterStateMustResolveToSignalObject=off  FilterRTWStateStorageClass=Auto  ParallelPVariant=InternalParameters  IdealPVariant=Disabled  IVariant=InternalParameters  DVariant=Disabled  IntegratorVariant=Continuous  SatVariant=Disabled  AWVariant=Passthrough  PCopyVariant=Disabled  TRVariant=Disabled  FdbkBlocksVariant=Forward  IdealPFdbkVariant=Disabled  SatFdbkVariant=Disabled  DerivativeFilterVariant=Disabled  NVariant=Disabled  NCopyVariant=Disabled_SignalSpec  FilterICVariant=Disabled  IntegratorICVariant=InternalICs  ExternalResetVariant=Disabled  TRSumVariant=Passthrough  SumFdbkVariant=Disabled  SumVariant=Sum_PI  TsampFilterVariant=InternalTs  TsampNgainVariant=Passthrough  TsampIntegralVariant=Passthrough  ExternalSaturationOutDataTypeStr=Inherit: Same as second input
  Step : Step  Commented=on  Time=1.2  After=10  SampleTime=0
  Step1 : Step  Commented=on  Time=0.3  After=10  SampleTime=0
  Step2 : Step  Commented=on  Time=0.5  After=10  SampleTime=0
  Step3 : Step  Commented=on  Time=0.6  After=15  SampleTime=0
  Step4 : Step  Commented=on  After=-10  SampleTime=0
  Step5 : Step  Commented=on  Time=1.7  After=-10  SampleTime=0
  Step6 : Step  Commented=on  Time=0.5  After=-10  SampleTime=0
  Step7 : Step  Commented=on  Time=0.8  After=-15  SampleTime=0
  wLdg->qg : Gain  Commented=on  Gain=500*pi*(L_Eingang_Shunt(1,1) +L_Ausgang_Shunt(1,1))
  wLdm->qm{,1..4} (5 alike) : Gain  Commented=on  Gain=400*pi*(L_Eingang_Shunt(1,1) +L_Ausgang_Shunt(1,1))
  wLqg->dg : Gain  Commented=on  Gain=500*pi*(L_Eingang_Shunt(1,1) +L_Ausgang_Shunt(1,1))
  wLqm->dm{,1..4} (5 alike) : Gain  Commented=on  Gain=400*pi*(L_Eingang_Shunt(1,1) +L_Ausgang_Shunt(1,1))
  Out1 : Outport
  Out2 : Outport  Port=2
  Out3 : Outport  Port=3
  Out4 : Outport  Port=4
  Out5 : Outport  Port=5
  Out6 : Outport  Port=6
  wires:
  Add9/1 -> PID Controller2/1
  Add10/1 -> PID Controller7/1
  [iq4] -> Add9/1, wLqm->dm/1
  Add12/1 -> PID Controller3/1
  [id5] -> Add13/2, wLdg->qg/1
  Add13/1 -> PID Controller1/1
  wLdm->qm/1 -> Gain3/1
  [id4] -> wLdm->qm/1, Add10/2
  wLqm->dm/1 -> Gain18/1
  Gain18/1 -> Add4/2
  Gain19/1 -> Add11/1
  PID Controller2/1 -> Add7/2
  PID Controller3/1 -> Add11/2
  PID Controller7/1 -> Add4/1
  wLdg->qg/1 -> Gain19/1
  PID Controller1/1 -> Add14/1
  [iq5] -> Add12/1, wLqg->dg/1
  wLqg->dg/1 -> Gain4/1
  In3/1 -> Bus Selector2/1
  Add1/1 -> Add9/2
  [id5_soll] -> Add2/1
  Step/1 -> Add1/2
  Add2/1 -> Add13/1
  Step1/1 -> Add2/2
  [iq4_soll] -> Add1/1
  Manual Switch/1 -> [id4_soll]
  Manual Switch1/1 -> [iq4_soll]
  Manual Switch2/1 -> [id5_soll]
  Manual Switch3/1 -> [iq5_soll]
  Constant/1 -> Manual Switch9/2, Manual Switch8/2, Manual Switch7/2, Manual Switch6/2, Manual Switch/2, Manual Switch5/2, Manual Switch4/2, Manual Switch1/2, Manual Switch2/2, Manual Switch3/2, Manual Switch10/2, Manual Switch11/2
  Add3/1 -> Add10/1
  Demux/1 -> [id4]
  Demux/2 -> [iq4]
  Demux1/1 -> [id5]
  Demux1/2 -> [iq5]
  Gain3/1 -> Add7/1
  Gain4/1 -> Add14/2
  [id4_soll] -> Add3/1
  Step2/1 -> Add3/2
  Add5/1 -> Add12/2
  [iq5_soll] -> Add5/3
  Step3/1 -> Add5/2
  Bus Selector2/2 -> Demux/1  "<idqp4_f>"
  Bus Selector2/3 -> Demux1/1  "<idqg5_f>"
  Constant3/1 -> Manual Switch3/1, Manual Switch9/1, Manual Switch10/1, Manual Switch11/1, Manual Switch8/1, Manual Switch7/1, Manual Switch6/1, Manual Switch2/1, Manual Switch1/1, Manual Switch/1, Manual Switch5/1, Manual Switch4/1
  In2/1 -> [theta]
  Mux11/1 -> First-Order Filter1/1
  Mux12/1 -> First-Order Filter2/1
  Step4/1 -> Add3/3
  Step5/1 -> Add1/3
  Step6/1 -> Add2/3
  Step7/1 -> Add5/1
  Add4/1 -> Mux11/1
  Add7/1 -> Mux11/2
  Add11/1 -> Mux12/2
  Add14/1 -> Mux12/1
  Bus Selector2/1 -> Demux4/1  "<idqg2_f>"
  Demux4/2 -> [iq2]
  Demux4/1 -> [id2]
  Bus Selector2/4 -> Demux5/1  "<idqp7_f>"
  Demux5/2 -> [iq7]
  Demux5/1 -> [id7]
  Bus Selector2/5 -> Demux6/1  "<idqg8_f>"
  Demux6/2 -> [iq8]
  Demux6/1 -> [id8]
  Demux7/1 -> [id19]
  Demux7/2 -> [iq19]
  Bus Selector2/6 -> Demux7/1  "<idqp19_f>"
  Manual Switch5/1 -> [iq2_soll]
  Manual Switch4/1 -> [id2_soll]
  Manual Switch7/1 -> [iq7_soll]
  Manual Switch6/1 -> [id7_soll]
  Manual Switch8/1 -> [id8_soll]
  Manual Switch9/1 -> [iq8_soll]
  Manual Switch11/1 -> [iq19_soll]
  Manual Switch10/1 -> [id19_soll]
  [id2_soll] -> Add6/1
  [id2] -> wLdm->qm1/1, Add6/2
  [iq2] -> Add8/1, wLqm->dm1/1
  [iq2_soll] -> Add8/2
  wLdm->qm1/1 -> Gain5/1
  wLqm->dm1/1 -> Gain6/1
  Add6/1 -> PID Controller4/1
  Add8/1 -> PID Controller5/1
  Gain6/1 -> Add15/2
  PID Controller4/1 -> Add15/1
  Gain5/1 -> Add16/1
  PID Controller5/1 -> Add16/2
  Add15/1 -> Gain7/1
  Add16/1 -> Gain8/1
  Gain7/1 -> Mux1/1
  Gain8/1 -> Mux1/2
  Mux1/1 -> First-Order Filter3/1
  First-Order Filter3/1 -> Out1/1
  First-Order Filter1/1 -> Out2/1
  First-Order Filter2/1 -> Out3/1
  Add17/1 -> Mux2/1
  [iq7_soll] -> Add20/2
  First-Order Filter4/1 -> Out4/1
  Gain10/1 -> Add17/2
  wLdm->qm2/1 -> Gain9/1
  PID Controller6/1 -> Add17/1
  Mux2/1 -> First-Order Filter4/1
  wLqm->dm2/1 -> Gain10/1
  [id7] -> wLdm->qm2/1, Add19/2
  Add18/1 -> Mux2/2
  Add20/1 -> PID Controller8/1
  Add19/1 -> PID Controller6/1
  Gain9/1 -> Add18/1
  PID Controller8/1 -> Add18/2
  [iq7] -> Add20/1, wLqm->dm2/1
  [id7_soll] -> Add19/1
  Add21/1 -> Mux3/1
  [iq8_soll] -> Add24/2
  First-Order Filter5/1 -> Out5/1
  Gain14/1 -> Add21/2
  wLdm->qm3/1 -> Gain13/1
  PID Controller9/1 -> Add21/1
  Mux3/1 -> First-Order Filter5/1
  wLqm->dm3/1 -> Gain14/1
  [id8] -> wLdm->qm3/1, Add23/2
  Add22/1 -> Mux3/2
  Add24/1 -> PID Controller10/1
  Add23/1 -> PID Controller9/1
  Gain13/1 -> Add22/1
  PID Controller10/1 -> Add22/2
  [iq8] -> Add24/1, wLqm->dm3/1
  [id8_soll] -> Add23/1
  Add25/1 -> Mux4/1
  [iq19_soll] -> Add28/2
  First-Order Filter6/1 -> Out6/1
  Gain22/1 -> Add25/2
  wLdm->qm4/1 -> Gain21/1
  PID Controller11/1 -> Add25/1
  Mux4/1 -> First-Order Filter6/1
  wLqm->dm4/1 -> Gain22/1
  [id19] -> wLdm->qm4/1, Add27/2
  Add26/1 -> Mux4/2
  Add28/1 -> PID Controller12/1
  Add27/1 -> PID Controller11/1
  Gain21/1 -> Add26/1
  PID Controller12/1 -> Add26/2
  [iq19] -> Add28/1, wLqm->dm4/1
  [id19_soll] -> Add27/1
